simulink model "simple_simulation"  (R2019b)
settings: Solver=VariableStepAuto  StartTime=0.0  StopTime=10.0  RelTol=1e-3
libraries: dspsrcs4 x1, simulink x1
settings Model: Creator=logan  LastModifiedBy=logan
settings SolverCC: AlgebraicLoopSolver=LineSearch
settings DataIOCC: ReturnWorkspaceOutputs=off
settings DebuggingCC: ModelReferenceExtraNoncontSigs=warning  ArithmeticOperatorsInVariantConditions=warning
settings SFSimCC: CustomCodeUndefinedFunction=UseInterfaceOnly

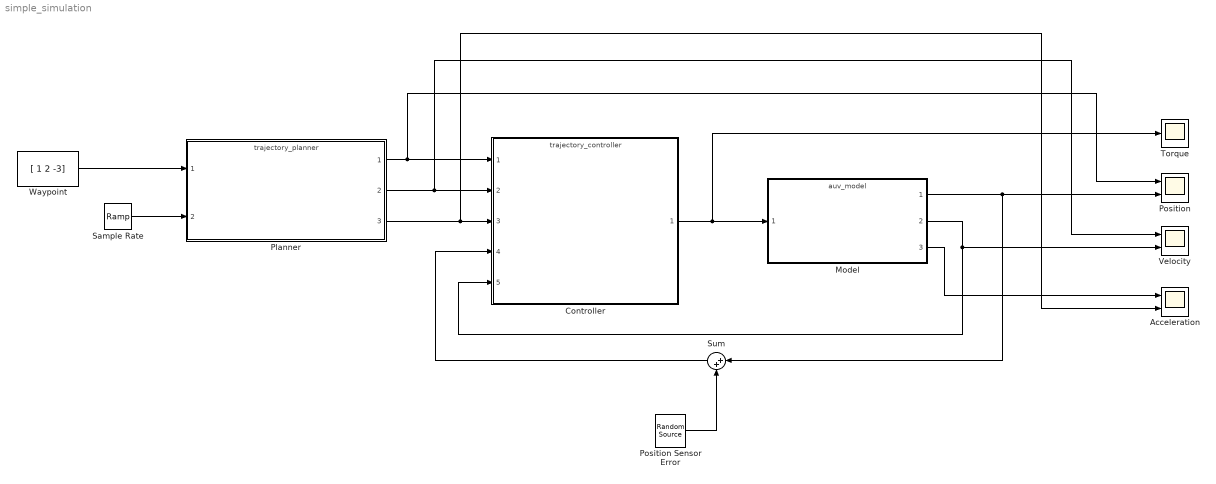
== system simple_simulation ==
  Acceleration : Scope  NumInputPorts=2
  Controller : ModelReference  ModelNameDialog=trajectory_controller.slx  SimulationMode=Normal  ModelReferenceVersion=1.8
  "Model " : ModelReference  ModelNameDialog=auv_model.slx  SimulationMode=Normal  ModelReferenceVersion=1.24
  Planner : ModelReference  ModelNameDialog=trajectory_planner.slx  SimulationMode=Normal  ModelReferenceVersion=1.14
  Position : Scope  NumInputPorts=2
  Position Sensor Error : dspsrcs4/Random Source  SrcType=Gaussian  NormMethod=Ziggurat  CltLength=12  MinVal=0  MaxVal=1  MeanVal=0  VarVal=1  RepMode=Not repeatable  rawSeed=1  IsInherit=off  SampMode=Discrete  SampTime=0.01  SampFrame=3  DataType=Double  OutComplex=Real  OutputFrames=off
  Sample Rate : simulink/Sources/Ramp  slope=1  start=0  InitialOutput=0
  Sum : Sum  Inputs=|++
  "Torque " : Scope
  Velocity : Scope  NumInputPorts=2
  Waypoint : Constant  Value=[ 1 2 -3]
  wires:
  Sample Rate/1 -> Planner/2
  Waypoint/1 -> Planner/1
  Planner/2 -> Velocity/1, Controller/2
  Planner/3 -> Acceleration/2, Controller/3
  Controller/1 -> "Torque "/1, "Model "/1
  "Model "/1 -> Sum/1, Position/2
  "Model "/2 -> Velocity/2, Controller/5
  Planner/1 -> Position/1, Controller/1
  Sum/1 -> Controller/4
  Position Sensor Error/1 -> Sum/2
  "Model "/3 -> Acceleration/1
